simulink model "linear_sim"  (R2025a)
settings: Solver=FixedStepAuto  StartTime=0.0  StopTime=30  FixedStep=dt_sim  RelTol=1e-3
values from neighbouring files (symbols this model uses):
  rA_hover = A_hover(4:end, 4:end)    [gain_scheduled_controller_design.m]
  rB_hover = B_hover(4:end, :)    [gain_scheduled_controller_design.m]
  rD_hover = zeros(9, 13)    [gain_scheduled_controller_design.m]
undefined symbols (not defined in the file or in its folder): Kr_hover, Kx_hover, ref_cmd_STEP
settings Model: Creator=alhallmark  LastModifiedBy=alhallmark

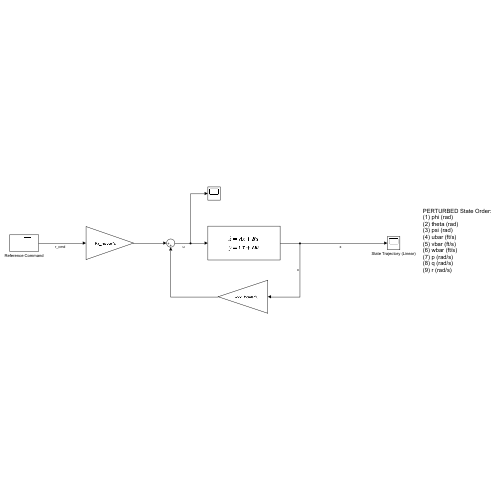
[thumbnail: Simulink's stored preview of the top-level diagram]
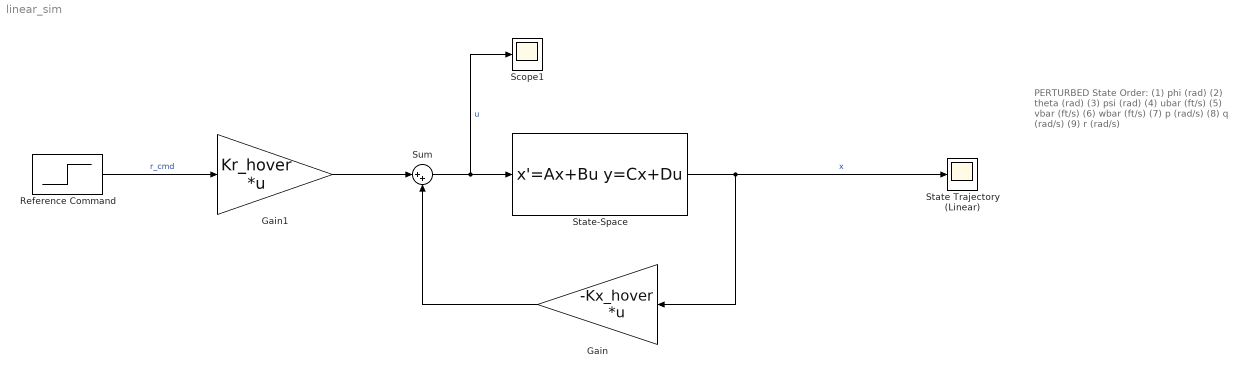
== system linear_sim ==
  note: PERTURBED State Order:
      | (1) phi (rad)
      | (2) theta (rad)
      | (3) psi (rad)
      | (4) ubar (ft/s)
      | (5) vbar (ft/s)
      | (6) wbar (ft/s)
      | (7) p (rad/s)
      | (8) q (rad/s)
      | (9) r (rad/s)
  Gain : Gain  Gain=-Kx_hover  Multiplication=Matrix(K*u)
  Gain1 : Gain  Gain=Kr_hover  Multiplication=Matrix(K*u)
  Reference Command : Step  Before=[0; 0; 0]  After=ref_cmd_STEP  SampleTime=0
  Scope1 : Scope
      settings: ActiveDisplayYMinimum=-1  ActiveDisplayYMaximum=1
  State Trajectory (Linear) : Scope
      settings: ActiveDisplayYMinimum=-0.71244302188533559  ActiveDisplayYMaximum=5.9286144079649432
  State-Space : StateSpace  A=rA_hover  B=rB_hover  C=eye(9)  D=rD_hover  InitialCondition=zeros(9,1)
  Sum : Sum  Inputs=|++
  wires:
  State-Space/1 -> State Trajectory (Linear)/1, Gain/1  "x"
  Sum/1 -> Scope1/1, State-Space/1  "u"
  Gain/1 -> Sum/2
  Gain1/1 -> Sum/1
  Reference Command/1 -> Gain1/1  "r_cmd"
